simulink model "Problem2_TrafficLightSystem"  (R2020b)
settings: Solver=VariableStepAuto  StartTime=0.0  StopTime=10.0  RelTol=1e-3
undefined symbols (not defined in the file): DiscIntNeverNeededParam
libraries: simulink x1
settings Model: Creator=vigne  LastModifiedBy=vigne

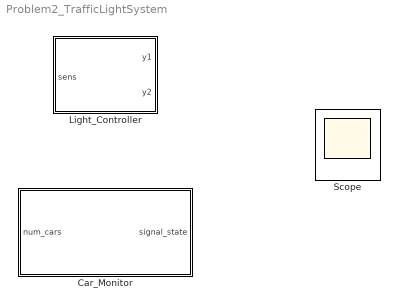
== system Problem2_TrafficLightSystem ==
  Car_Monitor : Subsystem
  Light_Controller : Stateflow chart  TreatAsAtomicUnit=on
  Scope : Scope  NumInputPorts=2

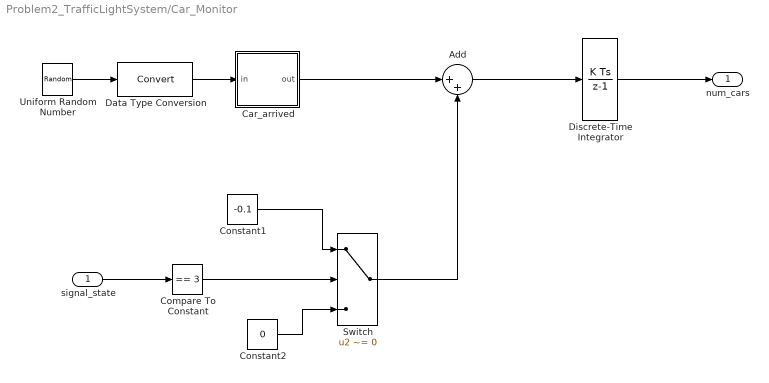
== system Problem2_TrafficLightSystem/Car_Monitor ==
  signal_state : Inport
  Add : Sum  Inputs=|++
  Car_arrived : Stateflow chart  TreatAsAtomicUnit=on
  Compare To Constant : simulink/Logic and Bit Operations/Compare To Constant  relop===  const=3  OutDataTypeStr=boolean  ZeroCross=off
  Constant1 : Constant  Value=-0.1
  Constant2 : Constant  Value=0
  Data Type Conversion : DataTypeConversion
  Discrete-Time Integrator : DiscreteIntegrator  SampleTime=-1  LimitOutput=on  LowerSaturationLimit=0  ICPrevOutput=DiscIntNeverNeededParam  ICPrevScaledInput=DiscIntNeverNeededParam
  Switch : Switch  Criteria=u2 ~= 0
  Uniform Random Number : UniformRandomNumber  Minimum=0  Maximum=100  Seed=177836  SampleTime=0
  num_cars : Outport  VectorParamsAs1DForOutWhenUnconnected=off
  wires:
  Uniform Random Number/1 -> Data Type Conversion/1
  Data Type Conversion/1 -> Car_arrived/1(in)
  Car_arrived/1(out) -> Add/1
  Add/1 -> Discrete-Time Integrator/1
  Switch/1 -> Add/2
  Compare To Constant/1 -> Switch/2
  signal_state/1 -> Compare To Constant/1
  Discrete-Time Integrator/1 -> num_cars/1
  Constant2/1 -> Switch/3
  Constant1/1 -> Switch/1

== stateflow chart Problem2_TrafficLightSystem/Light_Controller ==
  settings: stateMachineType=MOORE_MACHINE  executeAtInitialization=1  initializeOutput=1
  state Stop
    y1 = RED;
    y2 = GREEN;
  state StopForTraffic
    y1 = RED;
    y2 = GREEN;
  state StopToGo
    y1 = RED;
    y2 = YELLOW;
  state GoToStop
    y1 = YELLOW;
    y2 = RED;
  state Go
    y1 = GREEN;
    y2 = RED;
  (default) -> Stop
  StopForTraffic -> StopToGo : [sens]
  Stop -> StopForTraffic : after(20,tick)
  GoToStop -> Stop : after (3,tick)
  StopToGo -> Go : after(3,tick)
  Go -> GoToStop : after(10,tick)
  data: sens input double; y1 output double; RED constant uint8 =1; YELLOW constant double =2; GREEN constant double =3; y2 output double

== stateflow chart Problem2_TrafficLightSystem/Car_Monitor/Car_arrived ==
  (default) -> (junction 2) : {out = in > 98;}
  data: in input int8; out output double
